simulink model "Quadsim"  (R2012b)
settings: Solver=ode45  StartTime=0.0  StopTime=10.0  RelTol=1e-3
undefined symbols (not defined in the file): sigbuilder_block
settings Model: Creator=Estel  LastModifiedBy=Estel

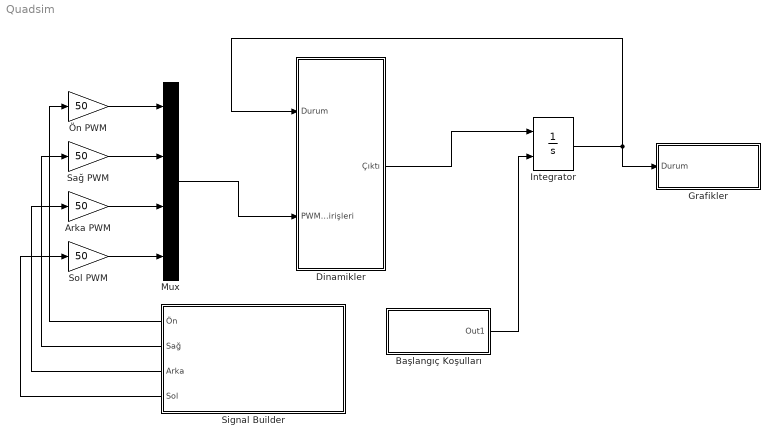
== system Quadsim ==
  Arka PWM : Gain  Gain=50
  Başlangıç Koşulları : Subsystem
  Dinamikler : Subsystem
  Grafikler : Subsystem
  Integrator : Integrator  InitialConditionSource=external
  Mux : Mux
  Sağ PWM : Gain  Gain=50
  Signal Builder : Subsystem  Tag=STV Subsys  LoadFcn=sigbuilder_block('load',[0 30 1024.5 489 ]);  StartFcn=sigbuilder_block('start');  StopFcn=sigbuilder_block('stop');  ClipboardFcn=sigbuilder_block('clipboard');  mask(Sigbuilder block){}
      mask help: Simulink:masks:SigbuilderBlock_MD
      mask init:
      | if ~strcmp(get_param(bdroot(gcbh),'SimulationStatus'),'stopped') tuvar = sigbuilder_block('maskInit'); end
      settings: CopyFcn=sigbuilder_block('copy');  DeleteFcn=sigbuilder_block('delete');  ModelCloseFcn=sigbuilder_block('modelClose');  PreSaveFcn=sigbuilder_block('preSave');  PauseFcn=sigbuilder_block('pause');  ContinueFcn=sigbuilder_block('continue');  NameChangeFcn=sigbuilder_block('namechange');  OpenFcn=sigbuilder_block('open',[6 28.5 1012.5 484.5 ]);  CloseFcn=sigbuilder_block('close');
      mask Display: plot(0, 0, 100, 100,[2, 2, 32, 32, 2], [68, 8, 8, 68, 68],[32, 2], [38, 38], [32, 19, 2],[53, 60, 44], [32, 17, 17, 2],[16, 16, 31, 31]);txt = getActiveGroup(gcbh);text(2, 100, txt,'verticalAlignment', 'top');
  Sol PWM : Gain  Gain=50
  Ön PWM : Gain  Gain=50
  wires:
  Signal Builder/4(Sol) -> Sol PWM/1
  Signal Builder/3(Arka) -> Arka PWM/1
  Signal Builder/2(Sağ) -> Sağ PWM/1
  Signal Builder/1(Ön) -> Ön PWM/1
  Arka PWM/1 -> Mux/3
  Sağ PWM/1 -> Mux/2
  Sol PWM/1 -> Mux/4
  Ön PWM/1 -> Mux/1
  Mux/1 -> Dinamikler/2(PWM Girişleri)
  Dinamikler/1(Çıktı) -> Integrator/1
  Integrator/1 -> Grafikler/1(Durum), Dinamikler/1(Durum)
  Başlangıç Koşulları/1(Out1) -> Integrator/2

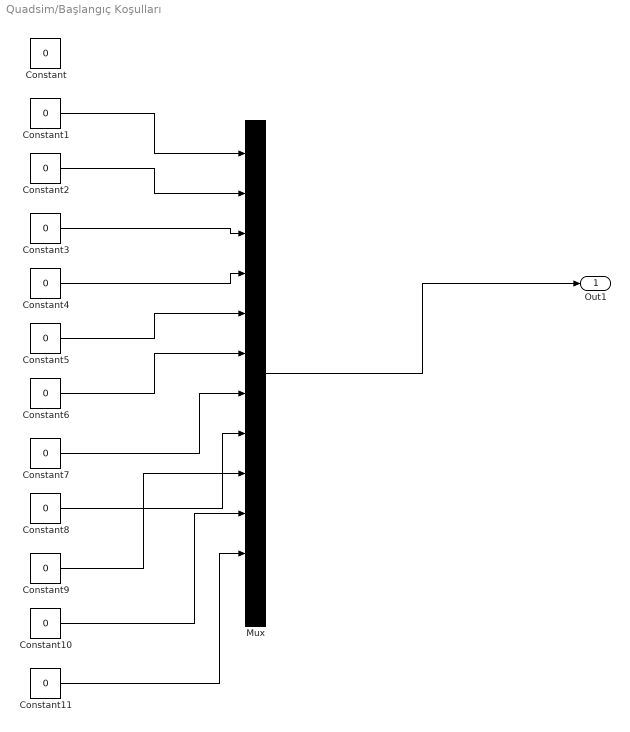
== system Quadsim/Başlangıç Koşulları ==
  Constant{,1..11} (12 alike) : Constant  Value=0
  Mux : Mux  Inputs=12
  Out1 : Outport
  wires:
  Constant3/1 -> Mux/3
  Constant4/1 -> Mux/4
  Constant5/1 -> Mux/5
  Constant2/1 -> Mux/2
  Constant6/1 -> Mux/6
  Constant1/1 -> Mux/1
  Constant7/1 -> Mux/7
  Constant8/1 -> Mux/8
  Constant9/1 -> Mux/9
  Constant10/1 -> Mux/10
  Constant11/1 -> Mux/11
  Mux/1 -> Out1/1

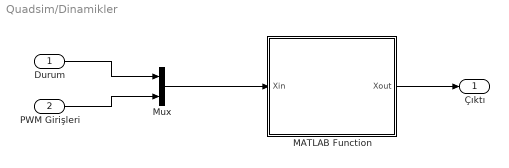
== system Quadsim/Dinamikler ==
  Durum : Inport
  PWM Girişleri : Inport  Port=2
  MATLAB Function : MATLAB Function  TreatAsAtomicUnit=on
  Mux : Mux  Inputs=2
  Çıktı : Outport
  wires:
  MATLAB Function/1(Xout) -> Çıktı/1
  PWM Girişleri/1 -> Mux/2
  Durum/1 -> Mux/1
  Mux/1 -> MATLAB Function/1(Xin)

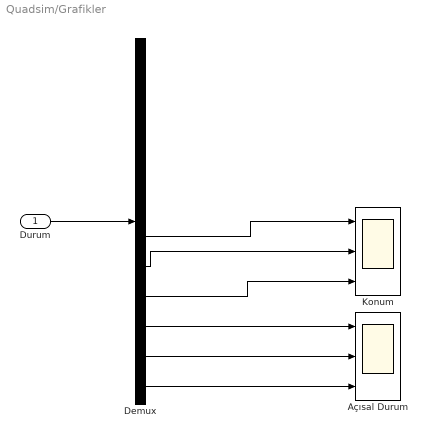
== system Quadsim/Grafikler ==
  Durum : Inport
  Açısal Durum : Scope  NumInputPorts=3
      settings: YMin=-5~-5~-5  YMax=5~5~5
  Demux : Demux  Outputs=12
  Konum : Scope  NumInputPorts=3
      settings: YMin=-5~-5~-5  YMax=5~5~5
  wires:
  Durum/1 -> Demux/1
  Demux/10 -> Açısal Durum/1
  Demux/11 -> Açısal Durum/2
  Demux/12 -> Açısal Durum/3
  Demux/7 -> Konum/1
  Demux/8 -> Konum/2
  Demux/9 -> Konum/3

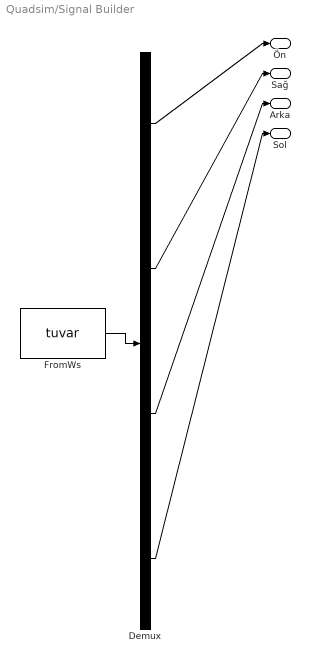
== system Quadsim/Signal Builder ==
  Demux : Demux  Tag=STV Demux
  FromWs : FromWorkspace  Tag=STV FromWs  VariableName=tuvar  SampleTime=0
      SigBuilderData=|
      | common.afterFinalStr = 'Extrapolate'
      | common.sampleTime = 0
      | dataSet.timeRange = [0 30]
      | dataSet.name = 'Group 1'
      | sbobj.Groups.Name = 'Group 1'
      | sbobj.Groups.Signals(1).Name = 'Ön'
      | sbobj.Groups.Signals(1).XData = [0 5 5 6 6 7 30]
      | sbobj.Groups.Signals(1).YData = [0.6 0.6 0.65 0.65 0.6 0.6 0.6]
      | sbobj.Groups.Signals(2).Name = 'Sağ'
      | sbobj.Groups.Signals(2).XData = [0 5 30]
      | sbobj.Groups.Signals(2).YData = [0.6 0.6 0.6]
      | sbobj.Groups.Signals(3).Name = 'Arka'
      | sbobj.Groups.Signals(3).XData = [0 5 5 6 6 7 30]
      | sbobj.Groups.Signals(3).YData = [0.6 0.6 0.55 0.55 0.6 0.6 0.6]
      | sbobj.Groups.Signals(4).Name = 'Sol'
      | sbobj.Groups.Signals(4).XData = [0 5 30]
      | sbobj.Groups.Signals(4).YData = [0.6 0.6 0.6]
      | sbobj.Groups.TimeRange = [0 30]
  Ön : Outport  Tag=STV Outport
  Sağ : Outport  Tag=STV Outport  Port=2
  Arka : Outport  Tag=STV Outport  Port=3
  Sol : Outport  Tag=STV Outport  Port=4
  wires:
  FromWs/1 -> Demux/1
  Demux/1 -> Ön/1
  Demux/2 -> Sağ/1
  Demux/3 -> Arka/1
  Demux/4 -> Sol/1

== matlab function Quadsim/Dinamikler/MATLAB Function ==
  data: Xout output; Xin input
function Xout   = quadrosim(Xin)

arm_l = 0.23;
craft_m = 0.65;
Ixx = 7.5*10^(-3);
Iyy = 7.5*10^(-3);
Izz = 1.3*10^(-2);
b = 3.13*10^(-5);  % Thrust factor
d = 7.5*10^(-7);  % Drag factor
g = 9.81;

% DURUM DEĞİŞKENLERİ
X_dot = Xin(1);
Y_dot = Xin(2);
Z_dot = Xin(3);
Roll_dot = Xin(4);
Pitch_dot = Xin(5);
Yaw_dot = Xin(6);
X = Xin(7);
Y = Xin(8);
Z = Xin(9);
Roll = Xin(10);
Pitch = Xin(11);
Yaw = Xin(12);
% X_dot1 = X_dot;
% Y_dot1 = Y_dot;
% Z_dot1 = Z_dot;
% Roll_dot1 = Roll_dot;
% Pitch_dot1 = Pitch_dot;
% Yaw_dot1 = Yaw_dot;

% % GİRDİLER
F = Xin(13);
R = Xin(14);
B = Xin(15);
L = Xin(16);

% İTKİ HESAPLARI
TF = b*F^2;
TR = b*R^2;
TB = b*B^2;
TL = b*L^2;
D = d*(-F+R-B+L);

% SİSTEM DİNAMİĞİ
% Model
% X_ddot = -(1/craft_m) * (cos(Roll)*sin(Pitch)*cos(Yaw) + sin(Roll)*sin(Yaw))*(TF+TR+TB+TL);
% Y_ddot = -(1/craft_m) * (cos(Roll)*sin(Pitch)*sin(Yaw) + sin(Roll)*cos(Yaw))*(TF+TR+TB+TL);
% z_craft_component = (1/craft_m)*cos(Roll)*cos(Pitch)*(TF+TR+TB+TL);
% Z_ddot = g - z_craft_component;
% Roll_ddot = Pitch_dot*Yaw_dot*(Iyy-Izz)/Ixx + ((arm_l)/Ixx)*(-TR+TL);
% Pitch_ddot = Roll_dot*Yaw_dot*(Izz-Ixx)/Iyy + ((arm_l)/Iyy)*(TF-TB);
% Yaw_ddot = Roll_dot*Pitch_dot*(Ixx-Iyy)/Izz + (D)/Izz;

% Basitleştirilmiş (Lineerize edilmiş) model
X_ddot = -(1/craft_m) * (cos(Roll)*sin(Pitch)*cos(Yaw) + sin(Roll)*sin(Yaw))*(TF+TR+TB+TL);
Y_ddot = -(1/craft_m) * (cos(Roll)*sin(Pitch)*sin(Yaw) + sin(Roll)*cos(Yaw))*(TF+TR+TB+TL);
z_craft_component = (1/craft_m)*cos(Roll)*cos(Pitch)*(TF+TR+TB+TL);
Z_ddot = -g + z_craft_component;
Roll_ddot = ((arm_l)/Ixx)*(-TR+TL);
Pitch_ddot = ((arm_l)/Iyy)*(TF-TB);
Yaw_ddot = (D)/Izz;

% ÇIKTI
Xout = [X_ddot Y_ddot Z_ddot Roll_ddot Pitch_ddot Yaw_ddot X_dot Y_dot Z_dot Roll_dot Pitch_dot Yaw_dot];

end
